simulink model "omnimorph_controller_FL_23"  (R2023b)
settings: Solver=ode1  StartTime=0.0  StopTime=inf  FixedStep=config.simVar.timeStep  RelTol=1e-3
undefined symbols (not defined in the file): Rx, Ry
libraries: robotcorelib x6, genomix x5, shareduavrstlib x4
settings Model: Creator=amr  LastModifiedBy=fiore
settings DataIOCC: ReturnWorkspaceOutputs=off
settings OptimizationCC: ReuseModelBlockBuffer=off
settings DebuggingCC: UnconnectedInputMsg=warning  UnconnectedOutputMsg=warning  UnconnectedLineMsg=warning  UnderSpecifiedDimensionMsg=warning
settings ModelReferenceCC: EnableRefExpFcnMdlSchedulingChecks=on
settings RTWCC: DLArmComputeVersion=19.05

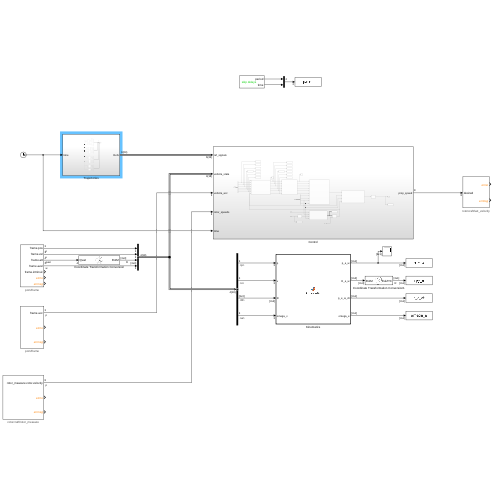
[thumbnail: Simulink's stored preview of the top-level diagram]
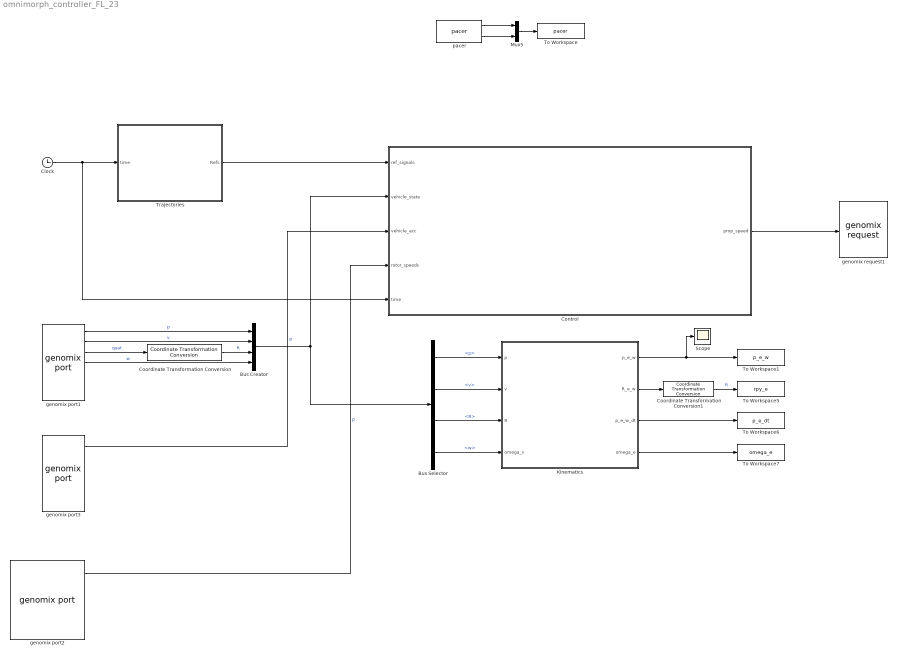
== system omnimorph_controller_FL_23 ==
  Bus Creator : BusCreator  Inputs=4
  Bus Selector : BusSelector  OutputSignals=p,v,R,w
  Clock : Clock
  Control : Subsystem
  Coordinate Transformation Conversion : robotcorelib/Coordinate Transformation Conversion  InputRepresentation=Quaternion  InputEulerSequence=ZYX  ShowTrVecInputPort=on  OutputRepresentation=Rotation Matrix  OutputEulerSequence=ZYX  ShowTrVecOutputPort=on  SimulateUsing=Interpreted execution
  Coordinate Transformation Conversion1 : robotcorelib/Coordinate Transformation Conversion  InputRepresentation=Rotation Matrix  InputEulerSequence=ZYX  ShowTrVecInputPort=on  OutputRepresentation=Euler Angles  OutputEulerSequence=ZYX  ShowTrVecOutputPort=on  SimulateUsing=Interpreted execution
  Kinematics : MATLAB Function  TreatAsAtomicUnit=on
  Mux5 : Mux  Inputs=2
  Scope : Scope
  To Workspace : ToWorkspace  VariableName=pacer  SaveFormat=Timeseries  SampleTime=-1
  To Workspace1 : ToWorkspace  VariableName=p_e_w  SampleTime=-1
  To Workspace5 : ToWorkspace  VariableName=rpy_e  SampleTime=-1
  To Workspace6 : ToWorkspace  VariableName=p_e_dt  SampleTime=-1
  To Workspace7 : ToWorkspace  VariableName=omega_e  SampleTime=-1
  Trajectories : Subsystem
  genomix port1 : genomix/genomix port  host=localhost  component=pom  port=frame  subport=robot  sigtype=value  timetype=periodic  period=config.simVar.timeStep  siglist="[{\"name\":\"frame.pos\",\"type\":\"value\",\"size\":3},{\"name\":\"frame.vel\",\"type\":\"value\",\"size\":3},{\"name\":\"frame.att\",\"type\":\"value\",\"size\":4},{\"name\":\"frame.avel\",\"type\":\"value\",\"size\":3},{\"name\":\"frame.intrinsic\",\"type\":\"value\",\"size\":1}]"
      settings: AttributesFormatString=pom/frame  SourceProductName=genomix
  genomix port2 : genomix/genomix port  host=localhost  component=rotorcraft  port=rotor_measure  sigtype=value  timetype=periodic  period=config.simVar.timeStep  siglist="[{\"name\":\"rotor_measure.rotor.velocity\",\"type\":\"value\",\"size\":8}]"
      settings: AttributesFormatString=rotorcraft/rotor_measure  SourceProductName=genomix
  genomix port3 : genomix/genomix port  host=localhost  component=pom  port=frame  subport=robot  sigtype=value  timetype=periodic  period=config.simVar.timeStep  siglist="[{\"name\":\"frame.acc\",\"type\":\"value\",\"size\":3}]"
      settings: AttributesFormatString=pom/frame  SourceProductName=genomix
  genomix request1 : genomix/genomix request  host=localhost  component=rotorcraft  port=set_velocity  sigtype=value  timetype=periodic  period=config.simVar.timeStep  siglist="[{\"name\":\"desired\",\"type\":\"value\",\"size\":8}]"
      settings: AttributesFormatString=rotorcraft/set_velocity  SourceProductName=genomix
  pacer : genomix/pacer  Priority=0  catchup=off
      settings: SourceProductName=genomix
  wires:
  Clock/1 -> Control/5(time), Trajectories/1(time)
  genomix port1/1 -> Bus Creator/1  "p"
  genomix port1/2 -> Bus Creator/2  "v"
  genomix port1/4 -> Bus Creator/4  "w"
  genomix port1/3 -> Coordinate Transformation Conversion/1  "quat"
  Coordinate Transformation Conversion/1 -> Bus Creator/3  "R"
  Bus Creator/1 -> Control/2(vehicle_state), Bus Selector/1
  Control/1(prop_speed) -> genomix request1/1
  pacer/2 -> Mux5/2
  pacer/1 -> Mux5/1
  Mux5/1 -> To Workspace/1
  genomix port3/1 -> Control/3(vehicle_acc)  "p"
  genomix port2/1 -> Control/4(rotor_speeds)  "p"
  Kinematics/3(p_e_w_dt) -> To Workspace6/1
  Kinematics/4(omega_e) -> To Workspace7/1
  Coordinate Transformation Conversion1/1 -> To Workspace5/1  "R"
  Kinematics/2(R_e_w) -> Coordinate Transformation Conversion1/1
  Bus Selector/1 -> Kinematics/1(p)  "<p>"
  Bus Selector/2 -> Kinematics/2(v)  "<v>"
  Bus Selector/3 -> Kinematics/3(R)  "<R>"
  Bus Selector/4 -> Kinematics/4(omega_v)  "<w>"
  Trajectories/1(Refs) -> Control/1(ref_signals)
  Kinematics/1(p_e_w) -> Scope/1, To Workspace1/1

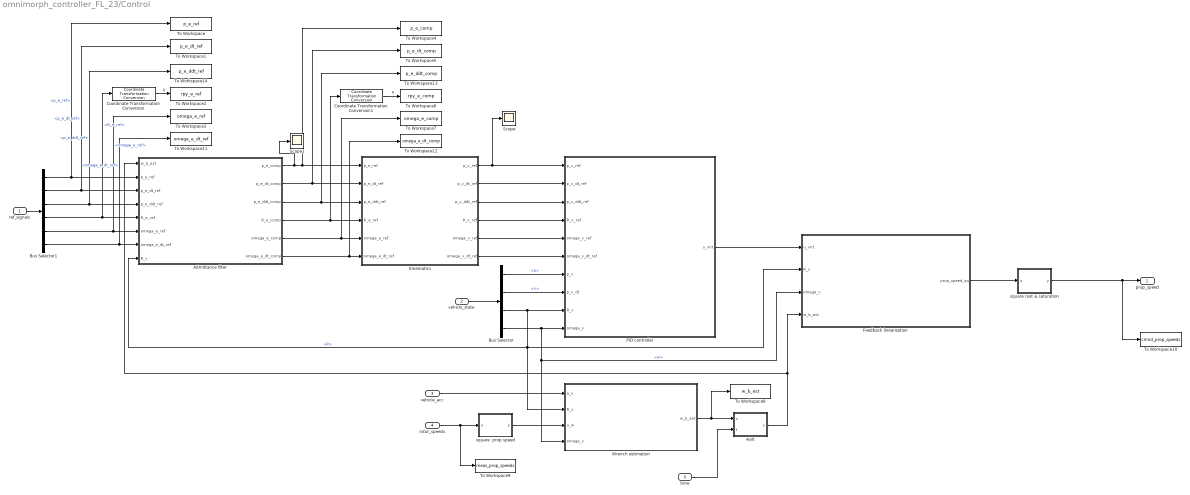
== system omnimorph_controller_FL_23/Control ==
  ref_signals : Inport
  vehicle_state : Inport  Port=2
  vehicle_acc : Inport  Port=3
  rotor_speeds : Inport  Port=4
  time : Inport  Port=5
  Admittance filter : Subsystem
  Bus Selector : BusSelector  OutputSignals=p,v,R,w
  Bus Selector1 : BusSelector  OutputSignals=p_e_ref,p_e_dt_ref,p_e_ddt_ref,R_e_ref,omega_e_ref,omega_e_dt_ref
  Coordinate Transformation Conversion : robotcorelib/Coordinate Transformation Conversion  InputRepresentation=Rotation Matrix  InputEulerSequence=ZYX  ShowTrVecInputPort=on  OutputRepresentation=Euler Angles  OutputEulerSequence=ZYX  ShowTrVecOutputPort=on  SimulateUsing=Interpreted execution
  Coordinate Transformation Conversion1 : robotcorelib/Coordinate Transformation Conversion  InputRepresentation=Rotation Matrix  InputEulerSequence=ZYX  ShowTrVecInputPort=on  OutputRepresentation=Euler Angles  OutputEulerSequence=ZYX  ShowTrVecOutputPort=on  SimulateUsing=Interpreted execution
  Feedback linearization : MATLAB Function  TreatAsAtomicUnit=on
  Kinematics : MATLAB Function  TreatAsAtomicUnit=on
  PID controller : MATLAB Function  TreatAsAtomicUnit=on
  Scope : Scope
  Scope1 : Scope
  To Workspace : ToWorkspace  VariableName=p_e_ref  SampleTime=-1
  To Workspace1 : ToWorkspace  VariableName=p_e_dt_ref  SampleTime=-1
  To Workspace10 : ToWorkspace  VariableName=cmnd_prop_speeds  SampleTime=-1
  To Workspace11 : ToWorkspace  VariableName=omega_e_dt_ref  SampleTime=-1
  To Workspace12 : ToWorkspace  VariableName=omega_e_dt_comp  SampleTime=-1
  To Workspace13 : ToWorkspace  VariableName=p_e_ddt_comp  SampleTime=-1
  To Workspace14 : ToWorkspace  VariableName=p_e_ddt_ref  SampleTime=-1
  To Workspace2 : ToWorkspace  VariableName=rpy_e_ref  SampleTime=-1
  To Workspace3 : ToWorkspace  VariableName=omega_e_ref  SampleTime=-1
  To Workspace4 : ToWorkspace  VariableName=p_e_comp  SampleTime=-1
  To Workspace5 : ToWorkspace  VariableName=p_e_dt_comp  SampleTime=-1
  To Workspace6 : ToWorkspace  VariableName=rpy_e_comp  SampleTime=-1
  To Workspace7 : ToWorkspace  VariableName=omega_e_comp  SampleTime=-1
  To Workspace8 : ToWorkspace  VariableName=w_b_est  SampleTime=-1
  To Workspace9 : ToWorkspace  VariableName=meas_prop_speeds  SampleTime=-1
  Wrench estimation : Subsystem
  square  prop speed : MATLAB Function  TreatAsAtomicUnit=on
  square root & saturation : MATLAB Function  TreatAsAtomicUnit=on
  wait : MATLAB Function  TreatAsAtomicUnit=on
  prop_speed : Outport
  wires:
  PID controller/1(u_virt) -> Feedback linearization/1(u_virt)
  Bus Selector/4 -> PID controller/10(omega_v), Wrench estimation/4(omega_v), Feedback linearization/3(omega_v)  "<w>"
  ref_signals/1 -> Bus Selector1/1
  square root & saturation/1(y) -> To Workspace10/1, prop_speed/1
  Admittance filter/1(p_e_comp) -> Scope1/1, To Workspace4/1, Kinematics/1(p_e_ref)
  Admittance filter/2(p_e_dt_comp) -> To Workspace5/1, Kinematics/2(p_e_dt_ref)
  Admittance filter/3(p_e_ddt_comp) -> To Workspace13/1, Kinematics/3(p_e_ddt_ref)
  Admittance filter/6(omega_e_dt_comp) -> To Workspace12/1, Kinematics/6(omega_e_dt_ref)
  Bus Selector1/6 -> To Workspace11/1, Admittance filter/7(omega_e_dt_ref)  "<omega_e_dt_ref>"
  Bus Selector1/5 -> To Workspace3/1, Admittance filter/6(omega_e_ref)  "<omega_e_ref>"
  Bus Selector1/4 -> Admittance filter/5(R_e_ref), Coordinate Transformation Conversion/1  "<R_e_ref>"
  Bus Selector1/3 -> To Workspace14/1, Admittance filter/4(p_e_ddt_ref)  "<p_e_ddt_ref>"
  Bus Selector1/2 -> To Workspace1/1, Admittance filter/3(p_e_dt_ref)  "<p_e_dt_ref>"
  Admittance filter/4(R_e_comp) -> Kinematics/4(R_e_ref), Coordinate Transformation Conversion1/1
  Kinematics/1(p_v_ref) -> Scope/1, PID controller/1(p_v_ref)
  Kinematics/2(p_v_dt_ref) -> PID controller/2(p_v_dt_ref)
  Kinematics/3(p_v_ddt_ref) -> PID controller/3(p_v_ddt_ref)
  Kinematics/5(omega_v_ref) -> PID controller/5(omega_v_ref)
  Kinematics/6(omega_v_dt_ref) -> PID controller/6(omega_v_dt_ref)
  Kinematics/4(R_v_ref) -> PID controller/4(R_v_ref)
  Admittance filter/5(omega_e_comp) -> Kinematics/5(omega_e_ref), To Workspace7/1
  Bus Selector/1 -> PID controller/7(p_v)  "<p>"
  Bus Selector/2 -> PID controller/8(p_v_dt)  "<v>"
  Bus Selector/3 -> Wrench estimation/2(R_v), Admittance filter/8(R_v), Feedback linearization/2(R_v), PID controller/9(R_v)  "<R>"
  Feedback linearization/1(prop_speed_sq) -> square root & saturation/1(u)
  vehicle_state/1 -> Bus Selector/1
  vehicle_acc/1 -> Wrench estimation/1(a_v)
  rotor_speeds/1 -> To Workspace9/1, square  prop speed/1(u)
  square  prop speed/1(y) -> Wrench estimation/3(u_w)
  wait/1(y) -> Admittance filter/1(w_b_ext), Feedback linearization/4(w_b_ext)
  time/1 -> wait/2(t)
  Bus Selector1/1 -> To Workspace/1, Admittance filter/2(p_e_ref)  "<p_e_ref>"
  Wrench estimation/1(w_b_ext) -> To Workspace8/1, wait/1(u)
  Coordinate Transformation Conversion/1 -> To Workspace2/1  "R"
  Coordinate Transformation Conversion1/1 -> To Workspace6/1  "R"

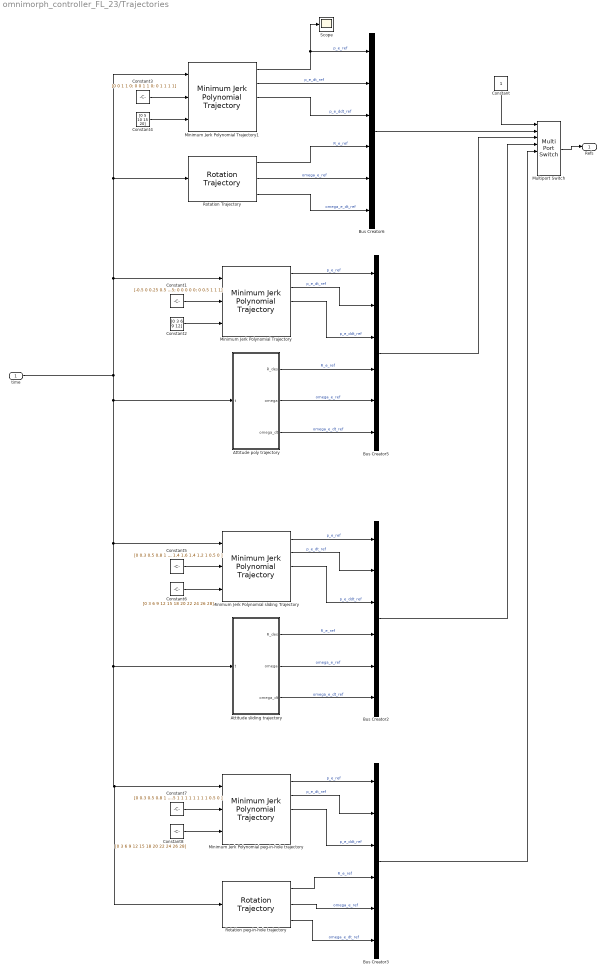
== system omnimorph_controller_FL_23/Trajectories ==
  time : Inport
  Attitude poly trajectory : MATLAB Function  TreatAsAtomicUnit=on
  Attitude sliding trajectory : MATLAB Function  TreatAsAtomicUnit=on
  Bus Creator{2..3,5..6} (4 alike) : BusCreator  Inputs=6
  Constant : Constant
  Constant1 : Constant  Value=[-0.5 0 0.25 0.5 0.5; 0 0 0 0 0; 0 0.5 1 1 1]
  Constant2 : Constant  Value=[0 3 6 9 12]
  Constant3 : Constant  Value=[0 0 1 1 0; 0 0 1 1 0; 0 1 1 1 1]
  Constant4 : Constant  Value=[0 5 10 15 20]
  Constant5 : Constant  Value=[0 0.3 0.5 0.8 1 1.2 1.2 1 0.8 0.5 0.3 0; 0 0 0 0 0 0 0 0 0 0 0 0; 0 0.5 1 1 1.2 1.4 1.6 1.4 1.2 1 0.5 0 ]
  Constant6 : Constant  Value=[0 3 6 9 12 15 18 20 22 24 26 28]
  Constant7 : Constant  Value=[0 0.3 0.5 0.8 1 1.2 1.4 1.2 1 0.8 0.5 0; 0 0 0 0 0 0 0 0 0 0 0 0; 0 0.5 1 1 1 1 1 1 1 1 0.5 0 ]
  Constant8 : Constant  Value=[0 3 6 9 12 15 18 20 22 24 26 28]
  Minimum Jerk Polynomial Trajectory : shareduavrstlib/Minimum Jerk Polynomial Trajectory  ShowBCInputPort=off  ShowPolynomialCoefs=off  ShowStatusOutputPort=off  TimeAllocation=off  TimeWeight=100  MinSegmentTime=0.1  MaxSegmentTime=1  MaxIteration=1500  MaxTime=10  SimulateUsing=Interpreted execution
      settings: LibrarySourceBlock=robotutilslib/Minimum Jerk Polynomial Trajectory
  Minimum Jerk Polynomial Trajectory1 : shareduavrstlib/Minimum Jerk Polynomial Trajectory  ShowBCInputPort=off  ShowPolynomialCoefs=off  ShowStatusOutputPort=off  TimeAllocation=off  TimeWeight=100  MinSegmentTime=0.1  MaxSegmentTime=1  MaxIteration=1500  MaxTime=10  SimulateUsing=Interpreted execution
      settings: LibrarySourceBlock=robotutilslib/Minimum Jerk Polynomial Trajectory
  Minimum Jerk Polynomial peg-in-hole trajectory : shareduavrstlib/Minimum Jerk Polynomial Trajectory  ShowBCInputPort=off  ShowPolynomialCoefs=off  ShowStatusOutputPort=off  TimeAllocation=off  TimeWeight=100  MinSegmentTime=0.1  MaxSegmentTime=1  MaxIteration=1500  MaxTime=10  SimulateUsing=Interpreted execution
      settings: LibrarySourceBlock=robotutilslib/Minimum Jerk Polynomial Trajectory
  Minimum Jerk Polynomial sliding Trajectory : shareduavrstlib/Minimum Jerk Polynomial Trajectory  ShowBCInputPort=off  ShowPolynomialCoefs=off  ShowStatusOutputPort=off  TimeAllocation=off  TimeWeight=100  MinSegmentTime=0.1  MaxSegmentTime=1  MaxIteration=1500  MaxTime=10  SimulateUsing=Interpreted execution
      settings: LibrarySourceBlock=robotutilslib/Minimum Jerk Polynomial Trajectory
  Multiport Switch : MultiPortSwitch  Inputs=7  SaturateOnIntegerOverflow=off  InputSameDT=off
  Rotation Trajectory : robotcorelib/Rotation Trajectory  WaypointFormat=Rotation Matrix  WaypointSource=Internal  R0=eye(3)  RF=Rx(pi)  TimeInterval=[ 5, 10 ]  CustomTimeScaling=off  ParameterSource=Internal  TSTime=0:0.1:1  TimeScaling=[ 0:0.1:1; ones( 1, 11 ); zeros( 1, 11 ) ]  SimulateUsing=Interpreted execution
      settings: LibrarySourceBlock=robotutilslib/Rotation Trajectory
  Rotation peg-in-hole trajectory : robotcorelib/Rotation Trajectory  WaypointFormat=Rotation Matrix  WaypointSource=Internal  R0=eye(3)  RF=Ry(pi/5)  TimeInterval=[ 5, 8 ]  CustomTimeScaling=off  ParameterSource=Internal  TSTime=0:0.1:1  TimeScaling=[ 0:0.1:1; ones( 1, 11 ); zeros( 1, 11 ) ]  SimulateUsing=Interpreted execution
      settings: LibrarySourceBlock=robotutilslib/Rotation Trajectory
  Scope : Scope
  Refs : Outport
  wires:
  Constant/1 -> Multiport Switch/1
  Constant1/1 -> Minimum Jerk Polynomial Trajectory/2
  Constant2/1 -> Minimum Jerk Polynomial Trajectory/3
  Minimum Jerk Polynomial Trajectory/1 -> Bus Creator5/1  "p_e_ref"
  Minimum Jerk Polynomial Trajectory/2 -> Bus Creator5/2  "p_e_dt_ref"
  Minimum Jerk Polynomial Trajectory/3 -> Bus Creator5/3  "p_e_ddt_ref"
  Attitude poly trajectory/2(omega) -> Bus Creator5/5  "omega_e_ref"
  Attitude poly trajectory/3(omega_dt) -> Bus Creator5/6  "omega_e_dt_ref"
  Attitude poly trajectory/1(R_des) -> Bus Creator5/4  "R_e_ref"
  Constant4/1 -> Minimum Jerk Polynomial Trajectory1/3
  Constant3/1 -> Minimum Jerk Polynomial Trajectory1/2
  Minimum Jerk Polynomial Trajectory1/1 -> Scope/1, Bus Creator6/1  "p_e_ref"
  Rotation Trajectory/1 -> Bus Creator6/4  "R_e_ref"
  Minimum Jerk Polynomial Trajectory1/2 -> Bus Creator6/2  "p_e_dt_ref"
  Minimum Jerk Polynomial Trajectory1/3 -> Bus Creator6/3  "p_e_ddt_ref"
  Rotation Trajectory/2 -> Bus Creator6/5  "omega_e_ref"
  Rotation Trajectory/3 -> Bus Creator6/6  "omega_e_dt_ref"
  Multiport Switch/1 -> Refs/1
  Bus Creator6/1 -> Multiport Switch/2
  Bus Creator5/1 -> Multiport Switch/3
  Minimum Jerk Polynomial sliding Trajectory/3 -> Bus Creator2/3  "p_e_ddt_ref"
  Minimum Jerk Polynomial sliding Trajectory/1 -> Bus Creator2/1  "p_e_ref"
  Minimum Jerk Polynomial sliding Trajectory/2 -> Bus Creator2/2  "p_e_dt_ref"
  Attitude sliding trajectory/2(omega) -> Bus Creator2/5  "omega_e_ref"
  Constant5/1 -> Minimum Jerk Polynomial sliding Trajectory/2
  Attitude sliding trajectory/3(omega_dt) -> Bus Creator2/6  "omega_e_dt_ref"
  Attitude sliding trajectory/1(R_des) -> Bus Creator2/4  "R_e_ref"
  Constant6/1 -> Minimum Jerk Polynomial sliding Trajectory/3
  Bus Creator2/1 -> Multiport Switch/4
  Constant8/1 -> Minimum Jerk Polynomial peg-in-hole trajectory/3
  Constant7/1 -> Minimum Jerk Polynomial peg-in-hole trajectory/2
  Minimum Jerk Polynomial peg-in-hole trajectory/3 -> Bus Creator3/3  "p_e_ddt_ref"
  Minimum Jerk Polynomial peg-in-hole trajectory/1 -> Bus Creator3/1  "p_e_ref"
  Minimum Jerk Polynomial peg-in-hole trajectory/2 -> Bus Creator3/2  "p_e_dt_ref"
  Rotation peg-in-hole trajectory/1 -> Bus Creator3/4  "R_e_ref"
  Rotation peg-in-hole trajectory/2 -> Bus Creator3/5  "omega_e_ref"
  Rotation peg-in-hole trajectory/3 -> Bus Creator3/6  "omega_e_dt_ref"
  Bus Creator3/1 -> Multiport Switch/5
  time/1 -> Minimum Jerk Polynomial Trajectory1/1, Rotation Trajectory/1, Minimum Jerk Polynomial Trajectory/1, Minimum Jerk Polynomial sliding Trajectory/1, Rotation peg-in-hole trajectory/1, Minimum Jerk Polynomial peg-in-hole trajectory/1, Attitude sliding trajectory/1(t), Attitude poly trajectory/1(t)

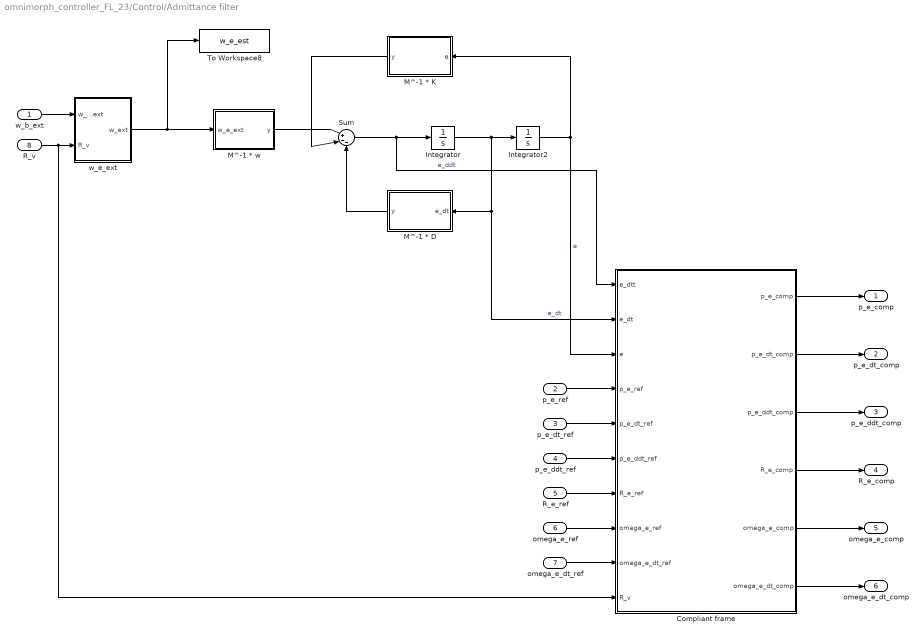
== system omnimorph_controller_FL_23/Control/Admittance filter ==
  w_b_ext : Inport
  p_e_ref : Inport  Port=2
  p_e_dt_ref : Inport  Port=3
  p_e_ddt_ref : Inport  Port=4
  R_e_ref : Inport  Port=5
  omega_e_ref : Inport  Port=6
  omega_e_dt_ref : Inport  Port=7
  R_v : Inport  Port=8
  Compliant frame : MATLAB Function  TreatAsAtomicUnit=on
  Integrator : Integrator
  Integrator2 : Integrator
  M^-1 * D : MATLAB Function  TreatAsAtomicUnit=on
  M^-1 * K : MATLAB Function  TreatAsAtomicUnit=on
  M^-1 * w : MATLAB Function  TreatAsAtomicUnit=on
  Sum : Sum  Inputs=|+--
  To Workspace8 : ToWorkspace  VariableName=w_e_est  SampleTime=-1
  w_e_ext : MATLAB Function  TreatAsAtomicUnit=on
  p_e_comp : Outport
  p_e_dt_comp : Outport  Port=2
  p_e_ddt_comp : Outport  Port=3
  R_e_comp : Outport  Port=4
  omega_e_comp : Outport  Port=5
  omega_e_dt_comp : Outport  Port=6
  wires:
  Integrator/1 -> Compliant frame/2(e_dt), M^-1 * D/1(e_dt), Integrator2/1  "e_dt"
  Sum/1 -> Compliant frame/1(e_dtt), Integrator/1  "e_ddt"
  M^-1 * K/1(y) -> Sum/2
  Integrator2/1 -> Compliant frame/3(e), M^-1 * K/1(e)  "e"
  M^-1 * D/1(y) -> Sum/3
  p_e_ref/1 -> Compliant frame/4(p_e_ref)
  p_e_dt_ref/1 -> Compliant frame/5(p_e_dt_ref)
  p_e_ddt_ref/1 -> Compliant frame/6(p_e_ddt_ref)
  R_e_ref/1 -> Compliant frame/7(R_e_ref)
  omega_e_ref/1 -> Compliant frame/8(omega_e_ref)
  omega_e_dt_ref/1 -> Compliant frame/9(omega_e_dt_ref)
  Compliant frame/6(omega_e_dt_comp) -> omega_e_dt_comp/1
  Compliant frame/5(omega_e_comp) -> omega_e_comp/1
  Compliant frame/4(R_e_comp) -> R_e_comp/1
  Compliant frame/3(p_e_ddt_comp) -> p_e_ddt_comp/1
  Compliant frame/2(p_e_dt_comp) -> p_e_dt_comp/1
  Compliant frame/1(p_e_comp) -> p_e_comp/1
  M^-1 * w/1(y) -> Sum/1
  w_b_ext/1 -> w_e_ext/1(w_b_ext)
  R_v/1 -> Compliant frame/10(R_v), w_e_ext/2(R_v)
  w_e_ext/1(w_ext) -> To Workspace8/1, M^-1 * w/1(w_e_ext)

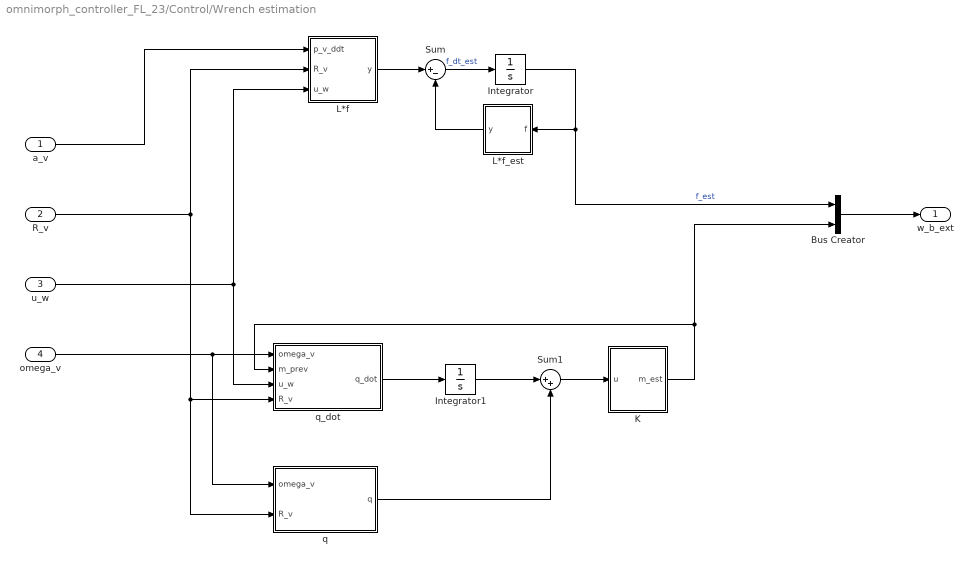
== system omnimorph_controller_FL_23/Control/Wrench estimation ==
  a_v : Inport
  R_v : Inport  Port=2
  u_w : Inport  Port=3
  omega_v : Inport  Port=4
  Bus Creator : BusCreator  Inputs=2
  Integrator : Integrator
  Integrator1 : Integrator
  K : MATLAB Function  TreatAsAtomicUnit=on
  L*f : MATLAB Function  TreatAsAtomicUnit=on
  L*f_est : MATLAB Function  TreatAsAtomicUnit=on
  Sum : Sum  Inputs=|+-
  Sum1 : Sum  Inputs=|++
  q : MATLAB Function  TreatAsAtomicUnit=on
  q_dot : MATLAB Function  TreatAsAtomicUnit=on
  w_b_ext : Outport
  wires:
  Sum/1 -> Integrator/1  "f_dt_est"
  Integrator/1 -> Bus Creator/1, L*f_est/1(f)  "f_est"
  L*f_est/1(y) -> Sum/2
  L*f/1(y) -> Sum/1
  R_v/1 -> q/2(R_v), q_dot/4(R_v), L*f/2(R_v)
  u_w/1 -> q_dot/3(u_w), L*f/3(u_w)
  omega_v/1 -> q/1(omega_v), q_dot/1(omega_v)
  a_v/1 -> L*f/1(p_v_ddt)
  Integrator1/1 -> Sum1/1
  q/1(q) -> Sum1/2
  Sum1/1 -> K/1(u)
  q_dot/1(q_dot) -> Integrator1/1
  Bus Creator/1 -> w_b_ext/1
  K/1(m_est) -> Bus Creator/2, q_dot/2(m_prev)

== matlab function omnimorph_controller_FL_23/Control/Admittance filter/M^-1 * w ==
  data: w_e_ext input; y output; config parameter
function y = fcn(w_e_ext,config)

M = config.conrtolParams.admitFilt.virtMass;
invM = diag([1/M(1,1);1/M(2,2);1/M(3,3);1/M(4,4);1/M(5,5);1/M(6,6)]);

y = invM*w_e_ext;

end

== matlab function omnimorph_controller_FL_23/Kinematics ==
  settings: updateMethod=DISCRETE
  data: p input; v input; R input; omega_v input; config parameter; p_e_w output; R_e_w output; p_e_w_dt output; omega_e output
function [p_e_w,R_e_w,p_e_w_dt,omega_e] = kinematic(p,v,R,omega_v,config)

p_e = config.uavParams.endEffector.p_e;
R_e = config.uavParams.endEffector.R_e;

p_e_w = p + R*p_e;
R_e_w = R*R_e;

omega_e = omega_v;
p_e_w_dt = v + skewMat(omega_v)*R*p_e;

end

== matlab function omnimorph_controller_FL_23/Trajectories/Attitude sliding trajectory ==
  data: R_des output; omega output; omega_dt output; t input; config parameter
function [R_des,omega,omega_dt] = fcn(t,config)

R = config.uavParams.endEffector.R_e; % R^B_E

R_des = R;
omega = [0;0;0];
omega_dt = [0;0;0];

end

== matlab function omnimorph_controller_FL_23/Control/Kinematics ==
  settings: updateMethod=DISCRETE
  data: p_e_ref input; p_e_dt_ref input; p_e_ddt_ref input; R_e_ref input; omega_e_ref input; omega_e_dt_ref input; config parameter; p_v_ref output; p_v_dt_ref output; p_v_ddt_ref output; R_v_ref output; omega_v_ref output; omega_v_dt_ref output
function [p_v_ref,p_v_dt_ref,p_v_ddt_ref,R_v_ref,omega_v_ref,omega_v_dt_ref] = kinematic(p_e_ref,p_e_dt_ref,p_e_ddt_ref,R_e_ref,omega_e_ref,omega_e_dt_ref,config)

p_e = config.uavParams.endEffector.p_e;
R_e = config.uavParams.endEffector.R_e;
%{
R_v_ref = R_e_ref*R_e.';
p_v_ref = p_e_ref - R_v_ref*p_e;

omega_v_ref = omega_e_ref;
p_v_dt_ref = p_e_dt_ref - R_v_ref*skewMat(omega_v_ref)*p_e;

omega_v_dt_ref = omega_e_dt_ref;
p_v_ddt_ref = p_e_ddt_ref - R_v_ref*skewMat(omega_v_dt_ref)*p_e - R_v_ref*skewMat(omega_v_ref)^2 *p_e;
%}

R_v_ref = R_e_ref*R_e.';
p_v_ref = p_e_ref - R_v_ref*p_e;

omega_v_ref = omega_e_ref;
p_v_dt_ref = p_e_dt_ref - skewMat(omega_v_ref)*R_v_ref*p_e;

omega_v_dt_ref = omega_e_dt_ref;
p_v_ddt_ref = p_e_ddt_ref - skewMat(omega_v_dt_ref)*R_v_ref*p_e - skewMat(omega_v_ref)^2 *R_v_ref*p_e;

end

== matlab function omnimorph_controller_FL_23/Control/Wrench estimation/L*f_est ==
  settings: updateMethod=DISCRETE
  data: f input; config parameter; y output
function y = fcn(f,config)

L = config.conrtolParams.wrenchObs.gains(1:3,1:3);
y = L*f;

end

== matlab function omnimorph_controller_FL_23/Control/Wrench estimation/L*f ==
  settings: updateMethod=DISCRETE
  data: p_v_ddt input; R_v input; u_w input; config parameter; y output
function y = fcn(p_v_ddt,R_v,u_w,config)

L = config.conrtolParams.wrenchObs.gains(1:3,1:3);
m = config.uavParams.mass;
g = config.gravity;
A = config.uavParams.wrenchMap;

f = m*p_v_ddt + m*g*[0;0;1] - R_v*A(1:3,:)*u_w;

y = L*f;

end

== matlab function omnimorph_controller_FL_23/Control/Wrench estimation/q_dot ==
  settings: updateMethod=DISCRETE
  data: omega_v input; m_prev input; u_w input; R_v input; config parameter; q_dot output size=[3 1]
function q_dot = fcn(omega_v,m_prev,u_w,R_v,config)

A = config.uavParams.wrenchMap;
J = config.uavParams.inertia;
omega_v_b = R_v'*omega_v; % Body frame angular velocity

q_dot = cross(omega_v_b,(J*omega_v_b)) - A(4:6,:)*u_w - m_prev;

end

== matlab function omnimorph_controller_FL_23/Control/Wrench estimation/q ==
  settings: updateMethod=DISCRETE
  data: omega_v input; R_v input; config parameter; q output
function q = fcn(omega_v,R_v,config)

J = config.uavParams.inertia;
omega_v_b = R_v'*omega_v; % Body frame angular velocity

% Assuming initial angular velocity is zero
q = J*omega_v_b;

end

== matlab function omnimorph_controller_FL_23/Control/Wrench estimation/K ==
  settings: updateMethod=DISCRETE
  data: u input; config parameter; m_est output
function m_est = fcn(u,config)

K = config.conrtolParams.wrenchObs.gains(4:6,4:6);
m_est = K*u;

end

== matlab function omnimorph_controller_FL_23/Control/Admittance filter/w_e_ext ==
  data: w_b_ext input; R_v input; w_ext output; config parameter
function w_ext = fcn(w_b_ext,R_v,config)

p_e = config.uavParams.endEffector.p_e;

H =  [eye(3),zeros(3);skewMat(R_v*p_e),eye(3)];
w_ext = H\[w_b_ext(1:3);R_v*w_b_ext(4:6)];

end

== matlab function omnimorph_controller_FL_23/Trajectories/Attitude poly trajectory ==
  data: R_des output; omega output; omega_dt output; t input; config parameter
function [R_des,omega,omega_dt] = fcn(t,config)

R = config.uavParams.endEffector.R_e; % R^B_E

R_des = R;
omega = [0;0;0];
omega_dt = [0;0;0];

end

== matlab function omnimorph_controller_FL_23/Control/square root & saturation ==
  data: u input; y output; config parameter
function y = fcn(u,config)   
    prop_max = config.uavParams.maxPropSpeed;
    prop_min = config.uavParams.minPropSpeed;

    y = sign(u) .* sqrt(abs(u));
    y = min(y, prop_max); % Clip positive values
    y = max(y, prop_min); % Clip negative values
end

== matlab function omnimorph_controller_FL_23/Control/PID controller ==
  settings: updateMethod=DISCRETE
  data: p_v_ref input; p_v_dt_ref input; p_v_ddt_ref input; R_v_ref input; omega_v_ref input; omega_v_dt_ref input; p_v input; p_v_dt input; R_v input; omega_v input; config parameter; u_virt output
function u_virt  = PIDPlus(p_v_ref,p_v_dt_ref,p_v_ddt_ref, ...
                                          R_v_ref,omega_v_ref,omega_v_dt_ref,...
                                          p_v,p_v_dt,...
                                          R_v,omega_v,config)

persistent eI_prev
        
if isempty(eI_prev)
    eI_prev = zeros(6,1);
end

%% initializations
u_virt = zeros(6,1);

Kp = config.conrtolParams.gainsPID.Kp;
Kv = config.conrtolParams.gainsPID.Kv;
KR = config.conrtolParams.gainsPID.KR;
Kw = config.conrtolParams.gainsPID.Kw;
KI_p = config.conrtolParams.gainsPID.KI_p;

dt = config.simVar.timeStep;

%% error signal computations 
ep =  p_v_ref - p_v;
ev = p_v_dt_ref - p_v_dt;
eI_p = eI_prev(1:3) + ep*dt;

eR = vmap(R_v_ref,R_v);
ew = R_v.' * (omega_v_ref - omega_v);
eI_R = eI_prev(4:6) + eR*dt;

eI_prev = [eI_p; eI_R];

%% compute u_virt
u_virt(1:3) = p_v_ddt_ref + Kv*ev + Kp*ep + KI_p*eI_p; 
u_virt(4:6) = omega_v_dt_ref + Kw*ew + KR*eR; 
end

== matlab function omnimorph_controller_FL_23/Control/Feedback linearization ==
  data: u_virt input size=[6, 1]; prop_speed_sq output size=[8,1]; R_v input size=[3, 3]; omega_v input; w_b_ext input size=[6 1]; config parameter
function prop_speed_sq = cntrl_FL(u_virt,R_v,omega_v,w_b_ext,config)

%% initializations
m = config.uavParams.mass; % uav mass
J = config.uavParams.inertia;%3x3 diag. uav Inertia mat.
A = config.uavParams.wrenchMap;
g = config.gravity;
omega_v_b = R_v'*omega_v; % Body frame angular velocity

J_inv = diag([1/J(1,1),1/J(2,2),1/J(3,3)]);
invInertia_mat = [eye(3)*(1/m), zeros(3); zeros(3),J_inv];
A_bar = invInertia_mat*[R_v, zeros(3); zeros(3), eye(3)]*A;
bias_forces = -[g*[0;0;1];J_inv*cross(omega_v_b,(J*omega_v_b))];
w_b = invInertia_mat*w_b_ext;

%% feedback linearization
prop_speed_sq = pinv(A_bar)*(-bias_forces + u_virt - w_b);

end

== matlab function omnimorph_controller_FL_23/Control/square  prop speed ==
  data: u input; y output
function y = fcn(u)
    y = sign(u) .* (abs(u).^2);
end

== matlab function omnimorph_controller_FL_23/Control/Admittance filter/M^-1 * K ==
  data: e input; y output; config parameter
function y = fcn(e,config)

K = config.conrtolParams.admitFilt.virtStiff;
M = config.conrtolParams.admitFilt.virtMass;
%invM = diag([1/M(1,1);1/M(2,2);1/M(3,3)]);
invM = diag([1/M(1,1);1/M(2,2);1/M(3,3);1/M(4,4);1/M(5,5);1/M(6,6)]);

y = invM*K*e;

end

== matlab function omnimorph_controller_FL_23/Control/wait ==
  data: u input; y output; t input
function y = fcn(u,t)

    if t<1.5
        y = [0;0;0;0;0;0];
    else
        y = u;
    end

end

== matlab function omnimorph_controller_FL_23/Control/Admittance filter/M^-1 * D ==
  data: e_dt input; y output; config parameter
function y = fcn(e_dt,config)

D = config.conrtolParams.admitFilt.virtDamp;
M = config.conrtolParams.admitFilt.virtMass;
%invM = diag([1/M(1,1);1/M(2,2);1/M(3,3)]);
invM = diag([1/M(1,1);1/M(2,2);1/M(3,3);1/M(4,4);1/M(5,5);1/M(6,6)]);

y = invM*D*e_dt;

end

== matlab function omnimorph_controller_FL_23/Control/Admittance filter/Compliant frame ==
  data: e_dtt input; e_dt input; e input; p_e_ref input; p_e_dt_ref input; p_e_ddt_ref input; R_e_ref input; omega_e_ref input; omega_e_dt_ref input; R_v input; p_e_comp output; config parameter; p_e_dt_comp output; p_e_ddt_comp output; R_e_comp output; omega_e_comp output; omega_e_dt_comp output
function [p_e_comp,p_e_dt_comp,p_e_ddt_comp,R_e_comp,omega_e_comp,omega_e_dt_comp] = fcn(e_dtt,e_dt,e,p_e_ref,p_e_dt_ref,p_e_ddt_ref, ...
                                                                                 R_e_ref,omega_e_ref,omega_e_dt_ref,R_v,config)
p_e_comp = p_e_ref + e(1:3);
p_e_dt_comp = p_e_dt_ref + e_dt(1:3);
p_e_ddt_comp = p_e_ddt_ref + e_dtt(1:3);

R_e_comp = (skewMat(e(4:6)) + eye(3))*R_e_ref;
omega_e_comp = omega_e_ref + e_dt(4:6);
omega_e_dt_comp = omega_e_dt_ref + e_dtt(4:6);
end
